simulink model "motor_model_w_load"  (R2015a)
settings: Solver=ode45  StartTime=0.0  StopTime=10.0  RelTol=1e-3
undefined symbols (not defined in the file or in its folder): Jm, kt, ra
settings Model: Creator=roevhat  LastModifiedBy=roevhat

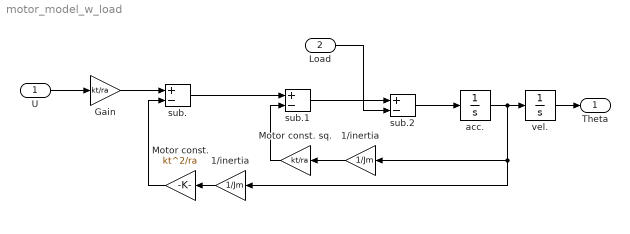
== system motor_model_w_load ==
  U : Inport
  Load : Inport  Port=2
  1/inertia : Gain  Gain=1/Jm
  "1/inertia " : Gain  Gain=1/Jm
  Gain : Gain  Gain=kt/ra
  Motor const. : Gain  Gain=kt^2/ra
  Motor const. sq. : Gain  Gain=kt/ra
  acc. : Integrator
  sub. : Sum  Inputs=+-
  sub.1 : Sum  Inputs=+-
  sub.2 : Sum  Inputs=+-
  vel. : Integrator
  Theta : Outport
  wires:
  U/1 -> Gain/1
  Gain/1 -> sub./1
  sub./1 -> sub.1/1
  Motor const./1 -> sub./2
  Motor const. sq./1 -> sub.1/2
  sub.1/1 -> sub.2/1
  sub.2/1 -> acc./1
  Load/1 -> sub.2/2
  "1/inertia "/1 -> Motor const. sq./1
  1/inertia/1 -> Motor const./1
  acc./1 -> 1/inertia/1, "1/inertia "/1, vel./1
  vel./1 -> Theta/1
